simulink model "SpheroMove_CVTInteg"  (R2013b)
settings: Solver=ode3  StartTime=0.0  StopTime=8  FixedStep=.1  RelTol=1e-3
InitFcn:
  | %sphName = uint8('Sphero-PGP');
  | 
  | %move(char(sphName), 0, 0)
StopFcn:
  | detectSpheroCVT( 10, 1);
  | 
  | %move(sphName, 0, 0)
  | %move(sphName, 0, 0, 0)
undefined symbols (not defined in the file or in its folder): IsPositionTracked, IsSkeletonTracked, JointDepthIndices, JointImageIndices, JointTrackingState, JointWorldCoordinates, none, PositionDepthIndices, PositionImageIndices, PositionWorldCoordinates, SegmentationData, SkeletonTrackingID, videoinput
libraries: visiontextngfix x1, imaqlib x1, utility x1, visionsinks x1
settings Model: Creator=dsethi  LastModifiedBy=dsethi
settings DataIOCC: SignalLoggingSaveFormat=ModelDataLogs
settings DebuggingCC: UnderspecifiedInitializationDetection=Simplified  MergeDetectMultiDrivingBlocksExec=error  MultiTaskDSMMsg=warning  MultiTaskCondExecSysMsg=none
settings RTWCC: IncludeERTFirstTime=on
settings GRTTargetCC: CodeReplacementLibrary=None  CPPClassGenCompliant=on

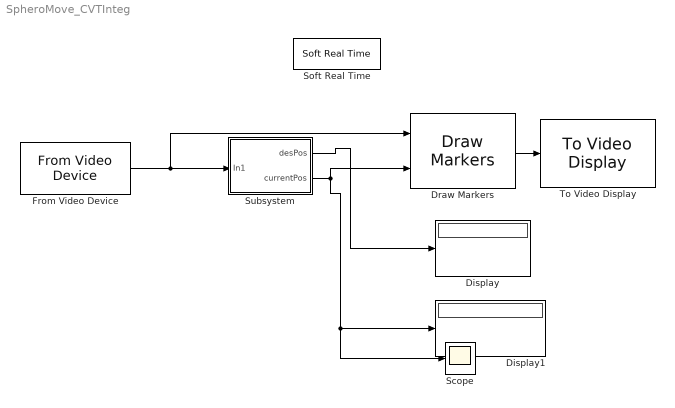
== system SpheroMove_CVTInteg ==
  Display : Display
  Display1 : Display
  Draw Markers : visiontextngfix/Draw Markers  shape=X-mark  size=3  fill=off  fillClrSource=Specify via dialog  display=User-specified value  intensity=200  color=[255 0 0]  opacity=0.6  viewport=Entire image  antialiasing=off  inType=Obsolete  imagePorts=One multidimensional signal  prodOutputMode=Binary point scaling  prodOutputWordLength=32  prodOutputFracLength=14  memoryMode=Specify word length  memoryWordLength=16  memoryFracLength=15  roundingMode=Floor  overflowMode=off
  From Video Device : imaqlib/From Video Device  DeviceMenu=winvideo 1 (Microsoft LifeCam Cinema)  Device=winvideo 1 (Microsoft LifeCam Cinema)  ObjConstructor=videoinput('winvideo', 1)  VideoFormatMenu=MJPG_640x360  VideoFormat=MJPG_640x360  VideoSource=input1  ROIPosition=[0 0 360 640]  EnableHWTrigger=off  TriggerConfiguration=none/none  SampleTime=0.1  OutputPortsMode=One multidimensional signal  DataType=single  CanDoHWTrigger=no  ReturnedColorSpace=rgb  BlockHandle=1921.0006  ROIWidth=640  ROIHeight=360  ROIColumn=0  ROIRow=0  EngXMLPath=C:\Program Files\MATLAB\R2013b\toolbox\imaq\imaq\private  DevXMLPath=C:\Program Files\MATLAB\R2013b\toolbox\imaq\imaqadaptors\win64  EngLibPath=C:\Program Files\MATLAB\R2013b\toolbox\imaq\imaqblks\imaqmex\win64  ColorSpace=rgb  BayerSensorAlignment=grbg  AllMetadata=IsPositionTracked;IsSkeletonTracked;JointDepthIndices;JointImageIndices;JointTrackingState;JointWorldCoordinates;PositionDepthIndices;PositionImageIndices;PositionWorldCoordinates;SegmentationData;SkeletonTrackingID
  Scope : Scope
      settings: SaveName=SpheroPos
  Soft Real Time : utility/Soft Real Time  x=1
  Subsystem : Subsystem  mask{cameraNum=Logitech, desPos=[200, 150]}
      mask prompts: cameraNum "Camera"; desPos "Desired position (x, y coordinates)"
      mask TypeOptions cameraNum: Logitech | Microsoft
  To Video Display : visionsinks/To Video Display  inputType=Obsolete  imagePorts=One multidimensional signal  OutputDevice=On-screen video monitor  fullScreen=off  videoWindowX=-7  videoWindowY=-5  saveWindowSize=off  videoWindowWidth=640  videoWindowHeight=360  dataOrg=Column-major  openAtMdlStart=on  isWindowOpen=off  inputColorFormat=RGB
  wires:
  Subsystem/1(desPos) -> Display/1
  Subsystem/2(currentPos) -> Scope/1, Display1/1, Draw Markers/2
  From Video Device/1 -> Draw Markers/1, Subsystem/1(In1)
  Draw Markers/1 -> To Video Display/1

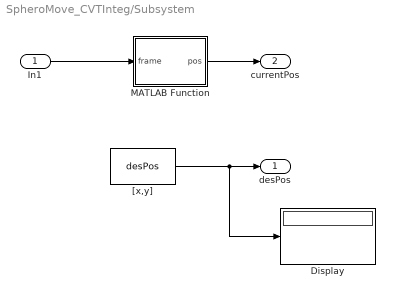
== system SpheroMove_CVTInteg/Subsystem ==
  In1 : Inport
  Display : Display
  MATLAB Function : MATLAB Function  TreatAsAtomicUnit=on
  "[x,y]" : Constant  Value=desPos
  desPos : Outport
  currentPos : Outport  Port=2
  wires:
  "[x,y]"/1 -> Display/1, desPos/1
  MATLAB Function/1(pos) -> currentPos/1
  In1/1 -> MATLAB Function/1(frame)

== matlab function SpheroMove_CVTInteg/Subsystem/Position tracking ==
  data: pos output; frame input
function pos = fcn(frame)
%#codegen
coder.extrinsic('detectSpheroCVT')
pos = [0; 0];

pos = detectSpheroCVT(frame);

== stateflow chart SpheroMove_CVTInteg/Chart ==
  state Control [parallel]
    settings: executionOrder=2
    state FindGains [parallel]
      settings: executionOrder=1
      state Outer
        en, du: Kp = 2;
        Ki = 0; Kd = 0;
      state Outermost
        en, du: Kp = 0.7;
        Ki = 0; Kd = 0;
      state Innermost
        en, du: Kp = 0;
        Ki = 0; Kd = 0;
      state Inner
        en, du: Kp = 4;
        Ki = 0; Kd = 0;
      (default) -> Outermost
      Outermost -> Outer : [dist<50]
      Outer -> Outermost [order 1] : [dist>=50]
      Inner -> Outer [order 1] : [dist>=30]
      Outer -> Inner [order 2] : [dist<30]
      Inner -> Innermost [order 2] : [dist<5]
      Innermost -> Inner : [dist>=5]
    state Motion [parallel]
      settings: executionOrder=2
      (default) -> (junction 27) : {speed = pid_control(dist, Kp, Ki, Kd)}
  state ComputeDist [parallel]
    en, du: [dist, angle] = relativePos(desPos, currPos)
    settings: executionOrder=1
  state u = pid_control(e,Kp,Ki,Kd) [function]
  data: desiredPos function_input; currentPos function_input; distance function_output; angleOut function_output; e function_input double size=1; u function_output; Kp function_input double size=1; Ki function_input double size=1; Kd function_input double size=1; speed output; dist local; angle output; desPos input; currPos input; Kp local; Ki local; Kd local
  function [distance, angleOut] = relativePos(desiredPos, currentPos):
    | function [distance, angleOut] = relativePos(desiredPos, currentPos)
    | 
    | coder.extrinsic('radtodeg', 'pdist')
    | 
    | if currPos(1)<0 || currPos(2)<0
    |     distance = Inf;
    |     angleOut = 0;
    |     return
    | end
    | %% Angle and distance calculation
    |  
    |     %Angle of desired position wrt y axis (or orientation of sphero)
    |     angleOut = atan2(desiredPos(1)-currentPos(1), desiredPos(2)-currentPos(2));
    | 
    |     if angleOut<0
    |         angleOut = -angleOut;
    |     else
    |         angleOut = 2*pi-angleOut;
    |     end
    | 
    |     angleOut = radtodeg(angleOut);
    | 
    |     distance = pdist([desiredPos'; currentPos']); %Distance or the error

== matlab function SpheroMove_CVTInteg/Sphero Move2 ==
  data: speed input; angle input; sphName parameter uint8
function fcn(speed, angle, sphName)
%#codegen
coder.extrinsic('move')

move(char(sphName), speed, angle);

== matlab function SpheroMove_CVTInteg/Subsystem/MATLAB Function ==
  data: frame input; pos output
function pos = fcn(frame)
%#codegen

coder.extrinsic('detectSpheroCVT')

pos = [0 0];

pos = detectSpheroCVT(frame);
